simulink model "demo"  (R2016a)
settings: Solver=FixedStepDiscrete  StartTime=0.0  StopTime=10  FixedStep=0.5  RelTol=1e-3
InitFcn:
  | k=0
undefined symbols (not defined in the file): serial
libraries: simulink_extras x4, instrumentlib x3
settings Model: Creator=11482  LastModifiedBy=11482

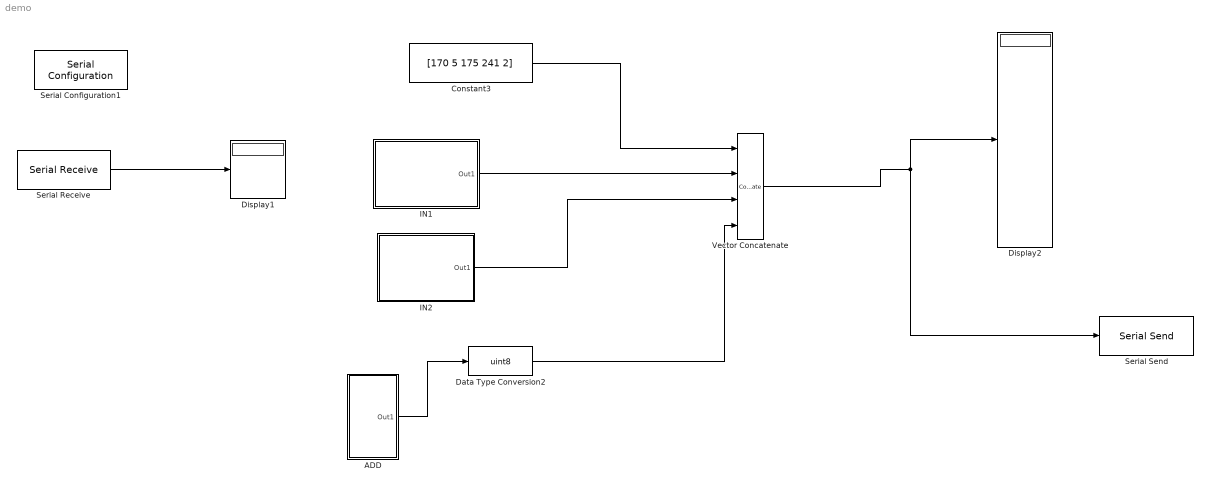
== system demo ==
  ADD : Subsystem
  Constant3 : Constant  Value=[170 5 175 241 2]  OutDataTypeStr=uint8  SampleTime=1
  Data Type Conversion2 : DataTypeConversion  OutDataTypeStr=uint8
  Display1 : Display
      settings: Format=hex (Stored Integer)
  Display2 : Display
      settings: Format=hex (Stored Integer)
  IN1 : Subsystem
  IN2 : Subsystem
  Serial Configuration1 : instrumentlib/Serial Configuration  Priority=-200000  ComPortMenu=COM3  ComPort=COM3  ObjConstructor=serial('COM3');  BaudRate=115200  DataBits=8  Parity=none  StopBits=1  FlowControl=none  Timeout=0.5  ByteOrder=BigEndian
  Serial Receive : instrumentlib/Serial Receive  ComPortMenu=<Please select a port...>  ComPort=COM3  ObjConstructor=serial('COM3');  Terminator=<none>  DataSize="[1  3]"  DataType=uint8  EnableBlockingMode=on  ActionDataUnavailable=Output last received value  CustomValue=0  SampleTime=1
  Serial Send : instrumentlib/Serial Send  ComPortMenu=COM3  ComPort=COM3  ObjConstructor=serial('COM3');  Terminator=<none>  EnableBlockingMode=on
  Vector Concatenate : Concatenate  NumInputs=4
  wires:
  Serial Receive/1 -> Display1/1
  Constant3/1 -> Vector Concatenate/1
  Vector Concatenate/1 -> Serial Send/1, Display2/1
  ADD/1(Out1) -> Data Type Conversion2/1
  Data Type Conversion2/1 -> Vector Concatenate/4
  IN1/1(Out1) -> Vector Concatenate/2
  IN2/1(Out1) -> Vector Concatenate/3

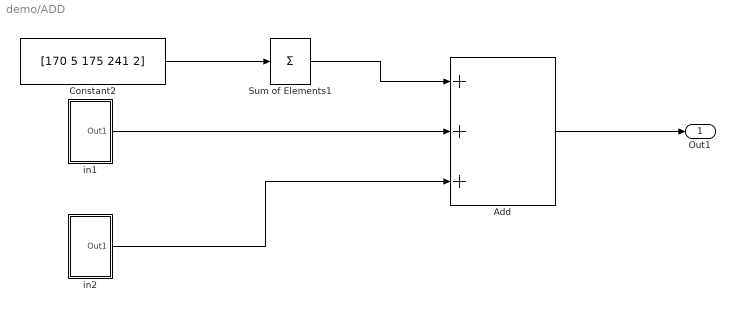
== system demo/ADD ==
  Add : Sum  Inputs=3  OutDataTypeStr=double
  Constant2 : Constant  Value=[170 5 175 241 2]  OutDataTypeStr=double
  Sum of Elements1 : Sum  Inputs=+  OutDataTypeStr=double
  in1 : Subsystem
  "in2 " : Subsystem
  Out1 : Outport
  wires:
  Constant2/1 -> Sum of Elements1/1
  Sum of Elements1/1 -> Add/1
  in1/1(Out1) -> Add/2
  "in2 "/1(Out1) -> Add/3
  Add/1 -> Out1/1

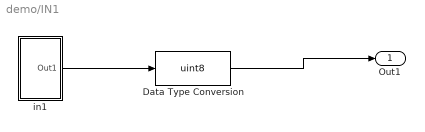
== system demo/IN1 ==
  Data Type Conversion : DataTypeConversion  OutDataTypeStr=uint8
  in1 : Subsystem
  Out1 : Outport
  wires:
  Data Type Conversion/1 -> Out1/1
  in1/1(Out1) -> Data Type Conversion/1

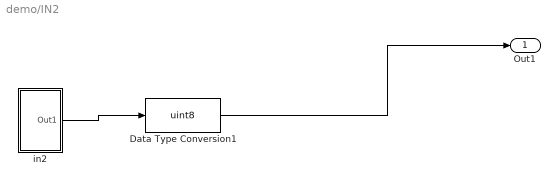
== system demo/IN2 ==
  Data Type Conversion1 : DataTypeConversion  OutDataTypeStr=uint8
  "in2 " : Subsystem
  Out1 : Outport
  wires:
  Data Type Conversion1/1 -> Out1/1
  "in2 "/1(Out1) -> Data Type Conversion1/1

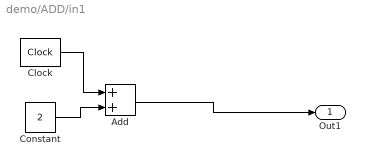
== system demo/ADD/in1 ==
  Add : Sum  Inputs=2  OutDataTypeStr=double
  Clock : simulink_extras/Flip Flops/Clock  period=2
  Constant : Constant  Value=2  OutDataTypeStr=double
  Out1 : Outport
  wires:
  Add/1 -> Out1/1
  Clock/1 -> Add/1
  Constant/1 -> Add/2

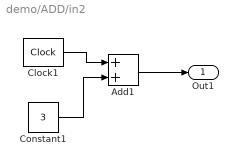
== system demo/ADD/in2  ==
  Add1 : Sum  Inputs=2  OutDataTypeStr=double
  Clock1 : simulink_extras/Flip Flops/Clock  period=2
  Constant1 : Constant  Value=3  OutDataTypeStr=double
  Out1 : Outport
  wires:
  Constant1/1 -> Add1/2
  Clock1/1 -> Add1/1
  Add1/1 -> Out1/1

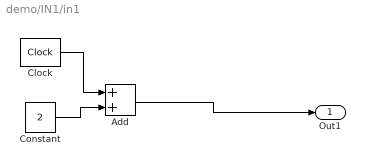
== system demo/IN1/in1 ==
  Add : Sum  Inputs=2  OutDataTypeStr=double
  Clock : simulink_extras/Flip Flops/Clock  period=2
  Constant : Constant  Value=2  OutDataTypeStr=double
  Out1 : Outport
  wires:
  Add/1 -> Out1/1
  Clock/1 -> Add/1
  Constant/1 -> Add/2

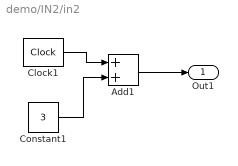
== system demo/IN2/in2  ==
  Add1 : Sum  Inputs=2  OutDataTypeStr=double
  Clock1 : simulink_extras/Flip Flops/Clock  period=2
  Constant1 : Constant  Value=3  OutDataTypeStr=double
  Out1 : Outport
  wires:
  Constant1/1 -> Add1/2
  Clock1/1 -> Add1/1
  Add1/1 -> Out1/1
